simulink model "translational_control_C1"  (R2016a)
settings: Solver=VariableStepAuto  StartTime=0.0  StopTime=10.0  RelTol=1e-3
undefined symbols (not defined in the file): tau_p, tau_v
settings Model: Creator=mgreiff  LastModifiedBy=mgreiff

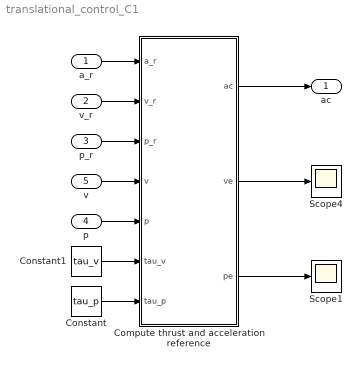
== system translational_control_C1 ==
  a_r : Inport  PortDimensions=3
  v_r : Inport  Port=2  PortDimensions=3
  p_r : Inport  Port=3  PortDimensions=3
  p : Inport  Port=4  PortDimensions=3
  v : Inport  Port=5  PortDimensions=3
  Compute thrust and acceleration reference : MATLAB Function  TreatAsAtomicUnit=on
  Constant : Constant  Value=tau_p
  Constant1 : Constant  Value=tau_v
  Scope1 : Scope
  Scope4 : Scope
  ac : Outport
  wires:
  a_r/1 -> Compute thrust and acceleration reference/1(a_r)
  p_r/1 -> Compute thrust and acceleration reference/3(p_r)
  Compute thrust and acceleration reference/1(ac) -> ac/1
  v_r/1 -> Compute thrust and acceleration reference/2(v_r)
  v/1 -> Compute thrust and acceleration reference/4(v)
  p/1 -> Compute thrust and acceleration reference/5(p)
  Compute thrust and acceleration reference/3(pe) -> Scope1/1
  Compute thrust and acceleration reference/2(ve) -> Scope4/1
  Constant1/1 -> Compute thrust and acceleration reference/6(tau_v)
  Constant/1 -> Compute thrust and acceleration reference/7(tau_p)

== matlab function translational_control_C1/Compute thrust and acceleration reference ==
  data: ac output; a_r input; v_r input; p_r input; v input; p input; ve output; pe output; tau_v input; tau_p input
function [ac, ve, pe] = C1(a_r,v_r,p_r,v,p, tau_v, tau_p)
    % ~~~~~~~~~ Copyright (c) 2018 Marcus Greiff (see LICENCE.md) ~~~~~~~~~
    %
    % Simple translational PD control in the global reference frame
    pe = 5*(p_r - p);
    ve = 5*(v_r - v);
    ac = a_r + (1/tau_v)*(ve) + (1/tau_p) * (pe);
end
